simulink model "control_design"  (R2025b)
settings: Solver=VariableStepAuto  StartTime=0.0  StopTime=10.0  RelTol=1e-3
libraries: slpidlib x2
settings Model: Creator=ken  LastModifiedBy=ken

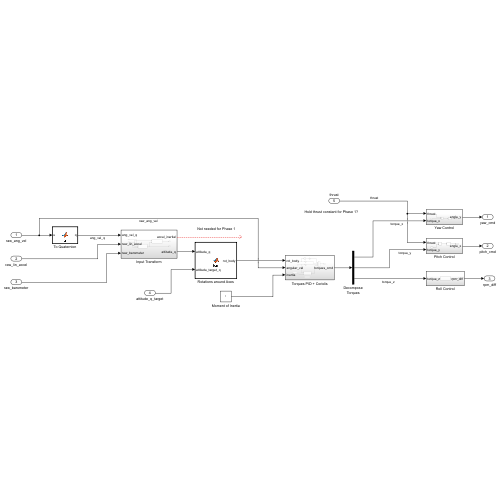
[thumbnail: Simulink's stored preview of the top-level diagram]
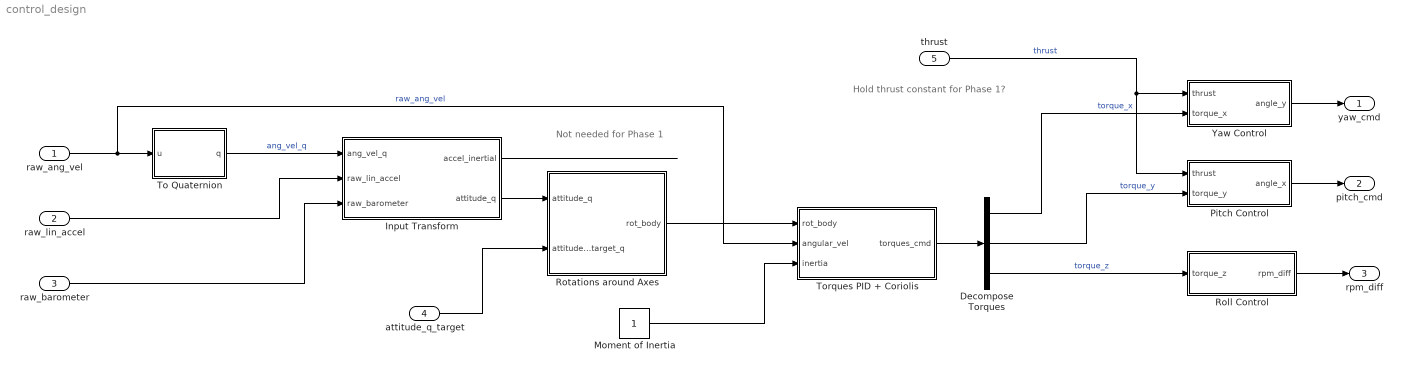
== system control_design ==
  note: Hold thrust constant for Phase 1?
  note: Not needed for Phase 1
  raw_ang_vel : Inport
  raw_lin_accel : Inport  Port=2
  raw_barometer : Inport  Port=3
  attitude_q_target : Inport  Port=4
  thrust : Inport  Port=5
  Decompose Torques : Demux  Outputs=3
  Input Transform : Subsystem
  Moment of Inertia : Constant
  Pitch Control : Subsystem
  Roll Control : Subsystem
  Rotations around Axes : MATLAB Function  TreatAsAtomicUnit=on
  To Quaternion : MATLAB Function  TreatAsAtomicUnit=on
  Torques PID + Coriolis : Subsystem
  Yaw Control : Subsystem
  yaw_cmd : Outport
  pitch_cmd : Outport  Port=2
  rpm_diff : Outport  Port=3
  wires:
  raw_lin_accel/1 -> Input Transform/2(raw_lin_accel)
  raw_ang_vel/1 -> Torques PID + Coriolis/2(angular_vel), To Quaternion/1(u)  "raw_ang_vel"
  raw_barometer/1 -> Input Transform/3(raw_barometer)
  Input Transform/2(attitude_q) -> Rotations around Axes/1(attitude_q)
  Rotations around Axes/1(rot_body) -> Torques PID + Coriolis/1(rot_body)
  To Quaternion/1(q) -> Input Transform/1(ang_vel_q)  "ang_vel_q"
  attitude_q_target/1 -> Rotations around Axes/2(attitude_target_q)
  Torques PID + Coriolis/1(torques_cmd) -> Decompose Torques/1
  Decompose Torques/2 -> Pitch Control/2(torque_y)  "torque_y"
  Decompose Torques/3 -> Roll Control/1(torque_z)  "torque_z"
  Moment of Inertia/1 -> Torques PID + Coriolis/3(inertia)
  Decompose Torques/1 -> Yaw Control/2(torque_x)  "torque_x"
  Input Transform/1(accel_inertial) -> ?
  thrust/1 -> Pitch Control/1(thrust), Yaw Control/1(thrust)  "thrust"
  Roll Control/1(rpm_diff) -> rpm_diff/1
  Yaw Control/1(angle_y) -> yaw_cmd/1
  Pitch Control/1(angle_x) -> pitch_cmd/1

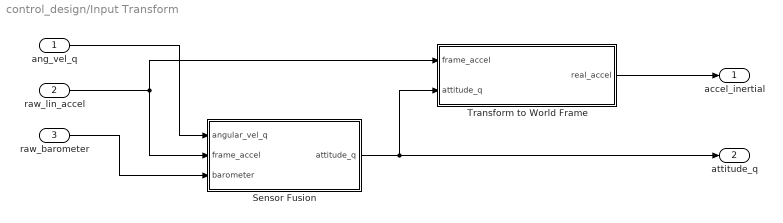
== system control_design/Input Transform ==
  ang_vel_q : Inport
  raw_lin_accel : Inport  Port=2
  raw_barometer : Inport  Port=3
  Sensor Fusion : MATLAB Function  TreatAsAtomicUnit=on
  Transform to World Frame : MATLAB Function  TreatAsAtomicUnit=on
  accel_inertial : Outport
  attitude_q : Outport  Port=2
  wires:
  ang_vel_q/1 -> Sensor Fusion/1(angular_vel_q)
  raw_lin_accel/1 -> Sensor Fusion/2(frame_accel), Transform to World Frame/1(frame_accel)
  raw_barometer/1 -> Sensor Fusion/3(barometer)
  Sensor Fusion/1(attitude_q) -> attitude_q/1, Transform to World Frame/2(attitude_q)
  Transform to World Frame/1(real_accel) -> accel_inertial/1

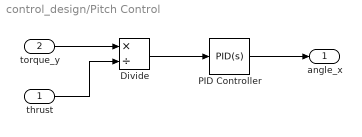
== system control_design/Pitch Control ==
  thrust : Inport
  torque_y : Inport  Port=2
  Divide : Product  Inputs=*/
  PID Controller : slpidlib/PID Controller  Controller=PID  Form=Parallel  TimeDomain=Continuous-time  UseExternalTs=off  SampleTime=-1  IntegratorMethod=Forward Euler  FilterMethod=Forward Euler  ControllerParametersSource=internal  P=1  I=1  UseKiTs=off  D=0  UseExternalDerivativeSource=off  N=100  UseFilter=on  TunerSelectOption=Transfer Function Based (PID Tuner App)  InitialConditionSource=internal  InitialConditionForIntegrator=0  InitialConditionForFilter=0  DifferentiatorICPrevScaledInput=0  ExternalReset=none  TrackingMode=off  Kt=1  LimitOutput=off  SatLimitsSource=internal  UpperSaturationLimit=inf  LowerSaturationLimit=-inf  LinearizeAsGain=on  AntiWindupMode=none  Kb=1  LimitIntegrator=off  UpperIntegratorSaturationLimit=inf  LowerIntegratorSaturationLimit=-inf  POutMin=[]  POutMax=[]  IOutMin=[]  IOutMax=[]  DOutMin=[]  DOutMax=[]  NOutMin=[]  NOutMax=[]  SumOutMin=[]  SumOutMax=[]  SaturationOutMin=[]  SaturationOutMax=[]  PParamMin=[]  PParamMax=[]  IParamMin=[]  IParamMax=[]  DParamMin=[]  DParamMax=[]  NParamMin=[]  NParamMax=[]  KbParamMin=[]  KbParamMax=[]  KtParamMin=[]  KtParamMax=[]  KbOutMin=[]  KbOutMax=[]  KtOutMin=[]  KtOutMax=[]  IntegratorOutMin=[]  IntegratorOutMax=[]  FilterOutMin=[]  FilterOutMax=[]  SumI1OutMin=[]  SumI1OutMax=[]  SumI2OutMin=[]  SumI2OutMax=[]  SumI3OutMin=[]  SumI3OutMax=[]  SumI4OutMin=[]  SumI4OutMax=[]  SumDOutMin=[]  SumDOutMax=[]  DifferentiatorOutMin=[]  DifferentiatorOutMax=[]  FilterDiffOutCoefMin=[]  FilterDiffOutCoefMax=[]  ReciprocalOutMin=[]  ReciprocalOutMax=[]  SumDenOutMin=[]  SumDenOutMax=[]  SumNumOutMin=[]  SumNumOutMax=[]  DivideOutMin=[]  DivideOutMax=[]  UdiffTsProdOutMin=[]  UdiffTsProdOutMax=[]  NTsProdOutMin=[]  NTsProdOutMax=[]  UintegralTsProdOutMin=[]  UintegralTsProdOutMax=[]  UngainTsProdOutMin=[]  UngainTsProdOutMax=[]  ClampingZeroOutDataTypeStr=Inherit: Inherit via back propagation  ClampingZeroOutMin=[]  ClampingZeroOutMax=[]  FilterDenConstantOutDataTypeStr=Inherit: Inherit via back propagation  FilterDenConstantOutMin=[]  FilterDenConstantOutMax=[]  PCopyOutDataTypeStr=Inherit: Inherit via back propagation  PCopyOutMin=[]  PCopyOutMax=[]  NCopyOutDataTypeStr=Inherit: Inherit via back propagation  NCopyOutMin=[]  NCopyOutMax=[]  IntegratorContinuousStateAttributes=''  IntegratorStateMustResolveToSignalObject=off  IntegratorRTWStateStorageClass=Auto  FilterContinuousStateAttributes=''  FilterStateMustResolveToSignalObject=off  FilterRTWStateStorageClass=Auto  ParallelPVariant=InternalParameters  IdealPVariant=Disabled  IVariant=InternalParameters  DVariant=InternalParameters  IntegratorVariant=Continuous  SatVariant=Disabled  AWVariant=Passthrough  PCopyVariant=Disabled  TRVariant=Disabled  FdbkBlocksVariant=Forward  IdealPFdbkVariant=Disabled  SatFdbkVariant=Disabled  DerivativeFilterVariant=ContFilter  NVariant=InternalParameters  NCopyVariant=Disabled  FilterICVariant=InternalICsFilter  IntegratorICVariant=InternalICs  ExternalResetVariant=Disabled  TRSumVariant=Passthrough  SumFdbkVariant=Disabled  SumVariant=Sum_PID  TsampFilterVariant=InternalTs  TsampNgainVariant=Passthrough  TsampIntegralVariant=Passthrough  ExternalSaturationOutDataTypeStr=Inherit: Same as second input  DerivativeSourceVariant=ErrorSignal  PreIntVariant=InternalPreInt
  angle_x : Outport
  wires:
  PID Controller/1 -> angle_x/1
  torque_y/1 -> Divide/1
  thrust/1 -> Divide/2
  Divide/1 -> PID Controller/1

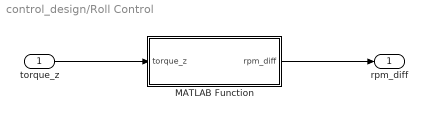
== system control_design/Roll Control ==
  torque_z : Inport
  MATLAB Function : MATLAB Function  TreatAsAtomicUnit=on
  rpm_diff : Outport
  wires:
  torque_z/1 -> MATLAB Function/1(torque_z)
  MATLAB Function/1(rpm_diff) -> rpm_diff/1

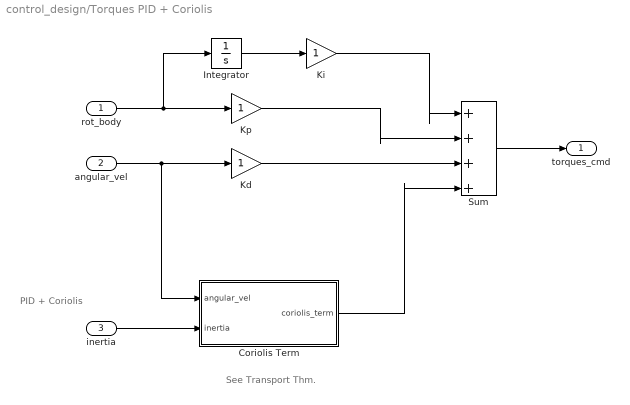
== system control_design/Torques PID + Coriolis ==
  note: See Transport Thm.
  note: PID + Coriolis
  rot_body : Inport
  angular_vel : Inport  Port=2
  inertia : Inport  Port=3
  Coriolis Term : MATLAB Function  TreatAsAtomicUnit=on
  Integrator : Integrator
  Kd : Gain
  Ki : Gain
  Kp : Gain
  Sum : Sum  Inputs=|+|+|+|+
  torques_cmd : Outport
  wires:
  rot_body/1 -> Kp/1, Integrator/1
  angular_vel/1 -> Coriolis Term/1(angular_vel), Kd/1
  Kd/1 -> Sum/3
  Kp/1 -> Sum/2
  Sum/1 -> torques_cmd/1
  Integrator/1 -> Ki/1
  Ki/1 -> Sum/1
  inertia/1 -> Coriolis Term/2(inertia)
  Coriolis Term/1(coriolis_term) -> Sum/4

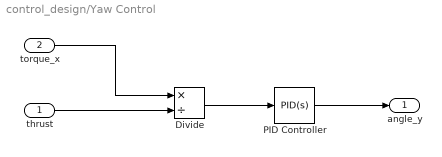
== system control_design/Yaw Control ==
  thrust : Inport
  torque_x : Inport  Port=2
  Divide : Product  Inputs=*/
  PID Controller : slpidlib/PID Controller  Controller=PID  Form=Parallel  TimeDomain=Continuous-time  UseExternalTs=off  SampleTime=-1  IntegratorMethod=Forward Euler  FilterMethod=Forward Euler  ControllerParametersSource=internal  P=1  I=1  UseKiTs=off  D=0  UseExternalDerivativeSource=off  N=100  UseFilter=on  TunerSelectOption=Transfer Function Based (PID Tuner App)  InitialConditionSource=internal  InitialConditionForIntegrator=0  InitialConditionForFilter=0  DifferentiatorICPrevScaledInput=0  ExternalReset=none  TrackingMode=off  Kt=1  LimitOutput=off  SatLimitsSource=internal  UpperSaturationLimit=inf  LowerSaturationLimit=-inf  LinearizeAsGain=on  AntiWindupMode=none  Kb=1  LimitIntegrator=off  UpperIntegratorSaturationLimit=inf  LowerIntegratorSaturationLimit=-inf  POutMin=[]  POutMax=[]  IOutMin=[]  IOutMax=[]  DOutMin=[]  DOutMax=[]  NOutMin=[]  NOutMax=[]  SumOutMin=[]  SumOutMax=[]  SaturationOutMin=[]  SaturationOutMax=[]  PParamMin=[]  PParamMax=[]  IParamMin=[]  IParamMax=[]  DParamMin=[]  DParamMax=[]  NParamMin=[]  NParamMax=[]  KbParamMin=[]  KbParamMax=[]  KtParamMin=[]  KtParamMax=[]  KbOutMin=[]  KbOutMax=[]  KtOutMin=[]  KtOutMax=[]  IntegratorOutMin=[]  IntegratorOutMax=[]  FilterOutMin=[]  FilterOutMax=[]  SumI1OutMin=[]  SumI1OutMax=[]  SumI2OutMin=[]  SumI2OutMax=[]  SumI3OutMin=[]  SumI3OutMax=[]  SumI4OutMin=[]  SumI4OutMax=[]  SumDOutMin=[]  SumDOutMax=[]  DifferentiatorOutMin=[]  DifferentiatorOutMax=[]  FilterDiffOutCoefMin=[]  FilterDiffOutCoefMax=[]  ReciprocalOutMin=[]  ReciprocalOutMax=[]  SumDenOutMin=[]  SumDenOutMax=[]  SumNumOutMin=[]  SumNumOutMax=[]  DivideOutMin=[]  DivideOutMax=[]  UdiffTsProdOutMin=[]  UdiffTsProdOutMax=[]  NTsProdOutMin=[]  NTsProdOutMax=[]  UintegralTsProdOutMin=[]  UintegralTsProdOutMax=[]  UngainTsProdOutMin=[]  UngainTsProdOutMax=[]  ClampingZeroOutDataTypeStr=Inherit: Inherit via back propagation  ClampingZeroOutMin=[]  ClampingZeroOutMax=[]  FilterDenConstantOutDataTypeStr=Inherit: Inherit via back propagation  FilterDenConstantOutMin=[]  FilterDenConstantOutMax=[]  PCopyOutDataTypeStr=Inherit: Inherit via back propagation  PCopyOutMin=[]  PCopyOutMax=[]  NCopyOutDataTypeStr=Inherit: Inherit via back propagation  NCopyOutMin=[]  NCopyOutMax=[]  IntegratorContinuousStateAttributes=''  IntegratorStateMustResolveToSignalObject=off  IntegratorRTWStateStorageClass=Auto  FilterContinuousStateAttributes=''  FilterStateMustResolveToSignalObject=off  FilterRTWStateStorageClass=Auto  ParallelPVariant=InternalParameters  IdealPVariant=Disabled  IVariant=InternalParameters  DVariant=InternalParameters  IntegratorVariant=Continuous  SatVariant=Disabled  AWVariant=Passthrough  PCopyVariant=Disabled  TRVariant=Disabled  FdbkBlocksVariant=Forward  IdealPFdbkVariant=Disabled  SatFdbkVariant=Disabled  DerivativeFilterVariant=ContFilter  NVariant=InternalParameters  NCopyVariant=Disabled  FilterICVariant=InternalICsFilter  IntegratorICVariant=InternalICs  ExternalResetVariant=Disabled  TRSumVariant=Passthrough  SumFdbkVariant=Disabled  SumVariant=Sum_PID  TsampFilterVariant=InternalTs  TsampNgainVariant=Passthrough  TsampIntegralVariant=Passthrough  ExternalSaturationOutDataTypeStr=Inherit: Same as second input  DerivativeSourceVariant=ErrorSignal  PreIntVariant=InternalPreInt
  angle_y : Outport
  wires:
  torque_x/1 -> Divide/1
  thrust/1 -> Divide/2
  Divide/1 -> PID Controller/1
  PID Controller/1 -> angle_y/1

== matlab function control_design/Input Transform/Sensor Fusion ==
  data: angular_vel_q input; attitude_q output; frame_accel input; barometer input
function attitude_q = fcn(angular_vel_q, frame_accel, barometer)

attitude_q = u;

end

== matlab function control_design/To Quaternion ==
  data: u input; q output
function q = fcn(u)

q = u;

== matlab function control_design/Rotations around Axes ==
  data: attitude_q input; attitude_target_q input; rot_body output
function rot_body = fcn(attitude_q, attitude_target_q)

rot_body = u;

== matlab function control_design/Torques PID + Coriolis/Coriolis Term ==
  data: angular_vel input; coriolis_term output; inertia input
function coriolis_term = fcn(angular_vel, inertia)

coriolis_term = u;

== matlab function control_design/Roll Control/MATLAB Function ==
  data: torque_z input; rpm_diff output
function rpm_diff = fcn(torque_z)

rpm_diff = u;

== matlab function control_design/Input Transform/Transform to World Frame ==
  data: frame_accel input; real_accel output; attitude_q input
function real_accel = fcn(frame_accel, attitude_q)

real_accel= u;
